simulink model "PMSM_Relay"  (R2014b)
settings: Solver=ode23tb  SolverMode=SingleTasking  StartTime=0.0  StopTime=0.1  RelTol=1e-4
libraries: powerlib x4
Description:
  | Copyright 2008-2014 The MathWorks, Inc.
settings Model: ExtModeTrigMode=oneshot  ExtModeArmWhenConnect=off  ExtModeAutoUpdateStatusClock=off  Creator=MathWorks  LastModifiedBy=Lei
settings DataIOCC: ExternalInput=[]  LimitDataPoints=off  SignalLoggingSaveFormat=ModelDataLogs  SaveOutput=off  SaveTime=off  SignalLoggingName=sigsOut
settings OptimizationCC: BlockReduction=off  BooleanDataType=off  ExpressionDepthLimit=2147483647  InitFltsAndDblsToZero=on  EfficientMapNaN2IntZero=off
settings DebuggingCC: UnderspecifiedInitializationDetection=Classic  MergeDetectMultiDrivingBlocksExec=none  CheckExecutionContextPreStartOutputMsg=on  CheckExecutionContextRuntimeOutputMsg=on  SignalResolutionControl=TryResolveAllWithWarning  SolverPrmCheckMsg=none  MultiTaskDSMMsg=warning  MultiTaskCondExecSysMsg=none  SigSpecEnsureSampleTimeMsg=none  FcnCallInpInsideContextMsg=UseLocalSettings  StateNameClashWarn=warning
settings HardwareCC: TargetUnknown=on
settings RTWCC: IncludeERTFirstTime=on
settings GRTTargetCC: CombineOutputUpdateFcns=off  GRTInterface=on

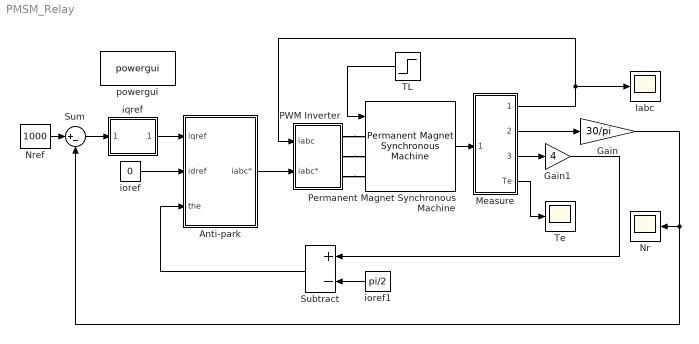
== system PMSM_Relay ==
  Anti-park : Subsystem
  Gain : Gain  Gain=30/pi  SaturateOnIntegerOverflow=on  OutDataTypeStr=Inherit: Same as input  ParamDataTypeStr=Inherit: Same as input
  Gain1 : Gain  Gain=4  SaturateOnIntegerOverflow=on  OutDataTypeStr=Inherit: Same as input  ParamDataTypeStr=Inherit: Same as input
  Iabc : Scope
      settings: TimeRange=0.06  YMin=-40  YMax=40  SaveName=Iabc
  Measure : Subsystem
  Nr : Scope
      settings: YMin=997.2  YMax=999.2  SaveName=Nr
  Nref : Constant  Value=1000
  PWM Inverter : Subsystem
  Permanent Magnet Synchronous Machine : powerlib/Machines/Permanent Magnet Synchronous Machine  NbPhases=3  FluxDistribution=Sinusoidal  RotorType=Salient-pole  MechanicalLoad=Torque Tm  PresetModel=No  ShowDetailedParameters=on  MeasurementBus=off  Resistance=2.875  Inductance=8.5e-3  dqInductances=[8.5e-3,8.5e-3]  La=0.00153  MachineConstant=Flux linkage established by magnets (V.s)  Flux=0.175  VoltageCst=126.966  TorqueCst=1.05  Flat=120  Mechanical=[0.8e-3, 0 4]  PolePairs=4  InitialConditions=[0,0, 0,0]  InitialConditions5ph=[0 0 0 0 0 0]  TsPowergui=0  TsBlock=-1  RefAngle=90 degrees behind phase A axis (modified Park)
  Subtract : Sum  Inputs=+-
  Sum : Sum  Inputs=|+-
  TL : Step  Time=0.05  Before=3  SampleTime=0
  "Te " : Scope
      settings: SaveName=Te
  ioref : Constant  Value=0
  ioref1 : Constant  Value=pi/2
  iqref : Subsystem  mask(PI Controller){I=0.06, P=1, sat=[-30, 30]}
      mask prompts: I "Integral"; P "Proportional:"; sat "Minimum and maximum outputs:"
      mask init:
      | min=sat(1);max=sat(2);
      mask Display: disp('PI')
  powergui : powerlib/powergui  SimulationMode=Continuous  SolverType=Tustin  SampleTime=0  frequency=60  SPID=on  DisableSnubberDevices=off  DisableRonSwitches=off  DisableVfSwitches=off  SwTol=0  DisplayEquations=off  Interpol=off  methode=off  Ts=0  frequencyindice=0  Pbase=100e6  ErrMax=1e-4  Iterations=50  UnitsV=kV  UnitsW=MW  FunctionMessages=off  echomessages=off  HookPort=off  EnableUseOfTLC=off  x0status=blocks  RestoreLinks=warning  ResistiveCurrentMeasurement=off  Frange=[0:2:500]  Ylog=off  Xlog=on  ShowGrid=off  save=off  variable=ZData  structure=0  ZoomFFT=on  StartTime=0.0  cycles=1  DisplayStyle=1  fundamental=60  FreqAxis=off  MaxFrequency=1000  frequencyindicesteady=1  RmsSteady=1  display=off
  wires:
  ioref/1 -> Anti-park/2(idref)
  Sum/1 -> iqref/1(In_1)
  Nref/1 -> Sum/1
  iqref/1(Out_1) -> Anti-park/1(iqref)
  Anti-park/1(iabc*) -> PWM Inverter/2(iabc*)
  Gain/1 -> Nr/1, Sum/2
  TL/1 -> Permanent Magnet Synchronous Machine/1
  Measure/1(Iabc) -> PWM Inverter/1(iabc), Iabc/1
  Permanent Magnet Synchronous Machine/1 -> Measure/1(In1)
  Measure/2(wm) -> Gain/1
  Measure/3(The) -> Gain1/1
  Measure/4(Te) -> "Te "/1
  ioref1/1 -> Subtract/2
  Gain1/1 -> Subtract/1
  Subtract/1 -> Anti-park/3(the)
  connections:
  PWM Inverter/RConn1 -- Permanent Magnet Synchronous Machine/LConn1
  PWM Inverter/RConn2 -- Permanent Magnet Synchronous Machine/LConn2
  PWM Inverter/RConn3 -- Permanent Magnet Synchronous Machine/LConn3

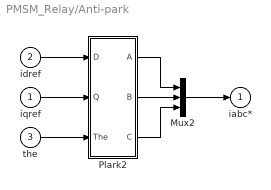
== system PMSM_Relay/Anti-park ==
  iqref : Inport
  idref : Inport  Port=2
  the : Inport  Port=3
  Mux2 : Mux  Inputs=3
  Plark2 : Subsystem
  iabc* : Outport  InitialOutput=0
  wires:
  the/1 -> Plark2/3(The)
  idref/1 -> Plark2/1(D)
  iqref/1 -> Plark2/2(Q)
  Plark2/2(B) -> Mux2/2
  Plark2/1(A) -> Mux2/1
  Plark2/3(C) -> Mux2/3
  Mux2/1 -> iabc*/1

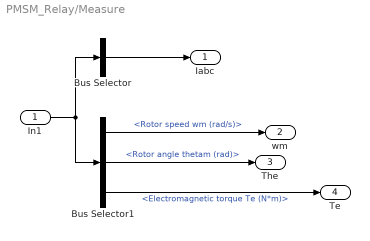
== system PMSM_Relay/Measure ==
  In1 : Inport
  Bus Selector : BusSelector  OutputSignals=Stator current is_a (A),Stator current is_b (A),Stator current is_c (A)  OutputAsBus=on
  Bus Selector1 : BusSelector  OutputSignals=Rotor speed wm (rad/s),Rotor angle thetam (rad),Electromagnetic torque Te (N*m)
  Iabc : Outport
  wm : Outport  Port=2
  The : Outport  Port=3
  Te : Outport  Port=4
  wires:
  Bus Selector1/1 -> wm/1  "<Rotor speed wm (rad/s)>"
  Bus Selector1/2 -> The/1  "<Rotor angle thetam (rad)>"
  Bus Selector/1 -> Iabc/1
  Bus Selector1/3 -> Te/1  "<Electromagnetic torque Te (N*m)>"
  In1/1 -> Bus Selector1/1, Bus Selector/1

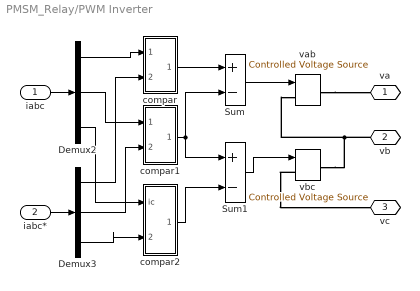
== system PMSM_Relay/PWM Inverter ==
  iabc : Inport
  iabc* : Inport  Port=2
  Demux2 : Demux  Outputs=3
  Demux3 : Demux  Outputs=3
  Sum : Sum  Inputs=+-  SaturateOnIntegerOverflow=on  InputSameDT=on  OutDataTypeStr=Inherit: Same as first input
  Sum1 : Sum  Inputs=+-  SaturateOnIntegerOverflow=on  InputSameDT=on  OutDataTypeStr=Inherit: Same as first input
  compar : Subsystem
  compar1 : Subsystem
  compar2 : Subsystem
  vab : powerlib/Electrical Sources/Controlled Voltage Source  Description=source block  Initialize=on  Source_Type=AC  Amplitude=0  Phase=0  Frequency=0  Measurements=None
      settings: AttributesFormatString=\n
  vbc : powerlib/Electrical Sources/Controlled Voltage Source  Description=source block  Initialize=on  Source_Type=AC  Amplitude=0  Phase=0  Frequency=0  Measurements=None
      settings: AttributesFormatString=\n
  va : PMIOPort  Port=1  Side=Right
  vb : PMIOPort  Port=2  Side=Right
  vc : PMIOPort  Port=3  Side=Right
  wires:
  Demux2/1 -> compar/1(ia)
  Demux2/2 -> compar1/1(ib)
  Demux2/3 -> compar2/1(ic)
  Demux3/3 -> compar2/2(ic*)
  Demux3/2 -> compar1/2(ib*)
  Demux3/1 -> compar/2(ia*)
  compar/1(va) -> Sum/1
  compar1/1(vb) -> Sum/2, Sum1/1
  compar2/1(vc) -> Sum1/2
  iabc/1 -> Demux2/1
  iabc*/1 -> Demux3/1
  Sum/1 -> vab/1
  Sum1/1 -> vbc/1
  connections:
  vab/RConn1 -- va/RConn1
  vb/RConn1 -- vbc/RConn1 -- vab/LConn1
  vbc/LConn1 -- vc/RConn1

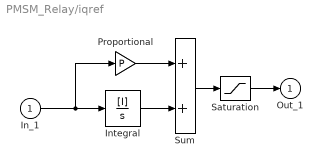
== system PMSM_Relay/iqref ==
  In_1 : Inport
  Integral : TransferFcn  Numerator=[I]  Denominator=[1 0]
  Proportional : Gain  Gain=P  SaturateOnIntegerOverflow=on  OutDataTypeStr=Inherit: Same as input  ParamDataTypeStr=Inherit: Same as input
  Saturation : Saturate  UpperLimit=max  LowerLimit=min
  Sum : Sum  SaturateOnIntegerOverflow=on  InputSameDT=on  OutDataTypeStr=Inherit: Same as first input
  Out_1 : Outport  InitialOutput=0
  wires:
  Integral/1 -> Sum/2
  In_1/1 -> Integral/1, Proportional/1
  Proportional/1 -> Sum/1
  Sum/1 -> Saturation/1
  Saturation/1 -> Out_1/1

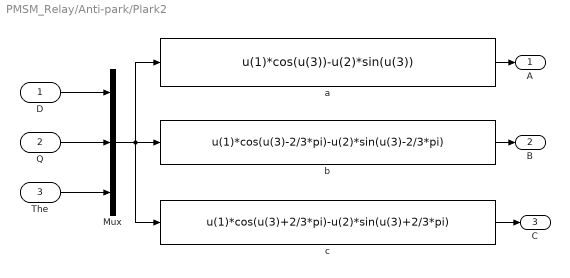
== system PMSM_Relay/Anti-park/Plark2 ==
  D : Inport
  Q : Inport  Port=2
  The : Inport  Port=3
  Mux : Mux  Inputs=3
  a : Fcn  Expr=u(1)*cos(u(3))-u(2)*sin(u(3))
  b : Fcn  Expr=u(1)*cos(u(3)-2/3*pi)-u(2)*sin(u(3)-2/3*pi)
  c : Fcn  Expr=u(1)*cos(u(3)+2/3*pi)-u(2)*sin(u(3)+2/3*pi)
  A : Outport
  B : Outport  Port=2
  C : Outport  Port=3
  wires:
  b/1 -> B/1
  The/1 -> Mux/3
  a/1 -> A/1
  D/1 -> Mux/1
  Q/1 -> Mux/2
  Mux/1 -> c/1, a/1, b/1
  c/1 -> C/1

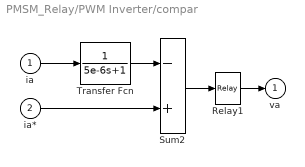
== system PMSM_Relay/PWM Inverter/compar ==
  ia : Inport
  ia* : Inport  Port=2
  Relay1 : Relay  OnSwitchValue=0.05  OffSwitchValue=-0.05  OnOutputValue=155  OffOutputValue=-155
  Sum2 : Sum  Inputs=-+  SaturateOnIntegerOverflow=on  InputSameDT=on  OutDataTypeStr=Inherit: Same as first input
  Transfer Fcn : TransferFcn  Denominator=[5e-6 1]
  va : Outport  InitialOutput=0
  wires:
  ia*/1 -> Sum2/2
  Sum2/1 -> Relay1/1
  Relay1/1 -> va/1
  ia/1 -> Transfer Fcn/1
  Transfer Fcn/1 -> Sum2/1

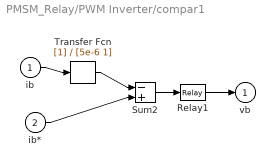
== system PMSM_Relay/PWM Inverter/compar1 ==
  ib : Inport
  ib* : Inport  Port=2
  Relay1 : Relay  OnSwitchValue=0.05  OffSwitchValue=-0.05  OnOutputValue=155  OffOutputValue=-155
  Sum2 : Sum  Inputs=-+  SaturateOnIntegerOverflow=on  InputSameDT=on  OutDataTypeStr=Inherit: Same as first input
  Transfer Fcn : TransferFcn  Denominator=[5e-6 1]
  vb : Outport  InitialOutput=0
  wires:
  ib*/1 -> Sum2/2
  Sum2/1 -> Relay1/1
  Relay1/1 -> vb/1
  ib/1 -> Transfer Fcn/1
  Transfer Fcn/1 -> Sum2/1

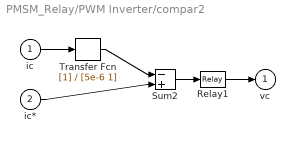
== system PMSM_Relay/PWM Inverter/compar2 ==
  ic : Inport
  ic* : Inport  Port=2
  Relay1 : Relay  OnSwitchValue=0.05  OffSwitchValue=-0.05  OnOutputValue=155  OffOutputValue=-155
  Sum2 : Sum  Inputs=-+  SaturateOnIntegerOverflow=on  InputSameDT=on  OutDataTypeStr=Inherit: Same as first input
  Transfer Fcn : TransferFcn  Denominator=[5e-6 1]
  vc : Outport  InitialOutput=0
  wires:
  ic*/1 -> Sum2/2
  Sum2/1 -> Relay1/1
  Relay1/1 -> vc/1
  ic/1 -> Transfer Fcn/1
  Transfer Fcn/1 -> Sum2/1
